simulink model "HW1_MealyV2"  (R2017a)
settings: Solver=VariableStepAuto  StartTime=0.0  StopTime=inf  RelTol=1e-3
settings Model: Creator=avise  LastModifiedBy=nauga

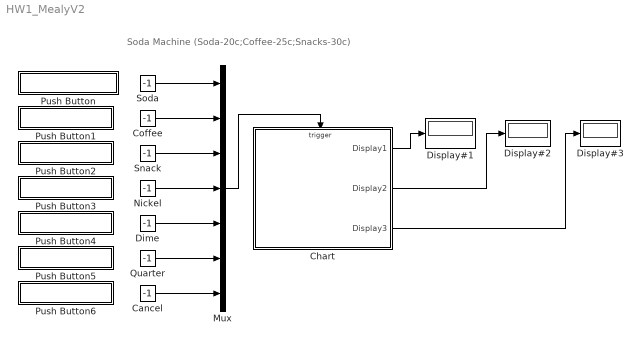
== system HW1_MealyV2 ==
  note: Soda Machine
      | (Soda-20c;Coffee-25c;Snacks-30c)
  Cancel : Constant  Value=-1
  Chart : Stateflow chart  TreatAsAtomicUnit=on
  Coffee : Constant  Value=-1
  Dime : Constant  Value=-1
  Display#1 : Display
  Display#2 : Display
  Display#3 : Display
  Mux : Mux  Inputs=7
  Nickel : Constant  Value=-1
  Push Button : Subsystem  DialogController=hmiCreateDDGDialog  IsWebBlock=on  mask(MWDashboardBlock){webBlockId=664f21db-061d-45c4-a5ed-301e6e3db717, webBlockType=pushbutton, ShowInLibBrwoser=on, ShowInitialText=on, HMISrcModelName=HW1_MealyV2}
      mask prompts: webBlockId "WebBlock Id"; webBlockType "WebBlock Type"; HMISrcModelName "Source Model"
      mask help: SimulinkHMI:dialogs:PushButtonDialogDesc
      mask Help: helpview([docroot '/mapfiles/simulink.map'], 'hmi_push_button')
      mask Display:
      | model = bdroot(gcb);
      | if strcmp(get_param(model,'BlockDiagramType'), 'library')
      |     image([(matlabroot) '/toolbox/simulink/hmi/icons/PushButton.png']);
      | end
  Push Button1 : Subsystem  DialogController=hmiCreateDDGDialog  IsWebBlock=on  mask(MWDashboardBlock){webBlockId=369ec6e0-de46-472e-8dd1-8918505b40b8, webBlockType=pushbutton, ShowInLibBrwoser=on, ShowInitialText=on, HMISrcModelName=HW1_MealyV2}
      mask prompts: webBlockId "WebBlock Id"; webBlockType "WebBlock Type"; HMISrcModelName "Source Model"
      mask help: SimulinkHMI:dialogs:PushButtonDialogDesc
      mask Help: helpview([docroot '/mapfiles/simulink.map'], 'hmi_push_button')
      mask Display:
      | model = bdroot(gcb);
      | if strcmp(get_param(model,'BlockDiagramType'), 'library')
      |     image([(matlabroot) '/toolbox/simulink/hmi/icons/PushButton.png']);
      | end
  Push Button2 : Subsystem  DialogController=hmiCreateDDGDialog  IsWebBlock=on  mask(MWDashboardBlock){webBlockId=437ecff1-f85d-43e6-a183-e5cb8b815949, webBlockType=pushbutton, ShowInLibBrwoser=on, ShowInitialText=on, HMISrcModelName=HW1_MealyV2}
      mask prompts: webBlockId "WebBlock Id"; webBlockType "WebBlock Type"; HMISrcModelName "Source Model"
      mask help: SimulinkHMI:dialogs:PushButtonDialogDesc
      mask Help: helpview([docroot '/mapfiles/simulink.map'], 'hmi_push_button')
      mask Display:
      | model = bdroot(gcb);
      | if strcmp(get_param(model,'BlockDiagramType'), 'library')
      |     image([(matlabroot) '/toolbox/simulink/hmi/icons/PushButton.png']);
      | end
  Push Button3 : Subsystem  DialogController=hmiCreateDDGDialog  IsWebBlock=on  mask(MWDashboardBlock){webBlockId=f2e822cd-a8a7-4ab8-9e8e-7b39c5c413d8, webBlockType=pushbutton, ShowInLibBrwoser=on, ShowInitialText=on, HMISrcModelName=HW1_MealyV2}
      mask prompts: webBlockId "WebBlock Id"; webBlockType "WebBlock Type"; HMISrcModelName "Source Model"
      mask help: SimulinkHMI:dialogs:PushButtonDialogDesc
      mask Help: helpview([docroot '/mapfiles/simulink.map'], 'hmi_push_button')
      mask Display:
      | model = bdroot(gcb);
      | if strcmp(get_param(model,'BlockDiagramType'), 'library')
      |     image([(matlabroot) '/toolbox/simulink/hmi/icons/PushButton.png']);
      | end
  Push Button4 : Subsystem  DialogController=hmiCreateDDGDialog  IsWebBlock=on  mask(MWDashboardBlock){webBlockId=f0c8a644-454f-4bf4-a778-a88d9125c533, webBlockType=pushbutton, ShowInLibBrwoser=on, ShowInitialText=on, HMISrcModelName=HW1_MealyV2}
      mask prompts: webBlockId "WebBlock Id"; webBlockType "WebBlock Type"; HMISrcModelName "Source Model"
      mask help: SimulinkHMI:dialogs:PushButtonDialogDesc
      mask Help: helpview([docroot '/mapfiles/simulink.map'], 'hmi_push_button')
      mask Display:
      | model = bdroot(gcb);
      | if strcmp(get_param(model,'BlockDiagramType'), 'library')
      |     image([(matlabroot) '/toolbox/simulink/hmi/icons/PushButton.png']);
      | end
  Push Button5 : Subsystem  DialogController=hmiCreateDDGDialog  IsWebBlock=on  mask(MWDashboardBlock){webBlockId=21d649ba-39b7-4048-9903-c8ade3fb44d4, webBlockType=pushbutton, ShowInLibBrwoser=on, ShowInitialText=on, HMISrcModelName=HW1_MealyV2}
      mask prompts: webBlockId "WebBlock Id"; webBlockType "WebBlock Type"; HMISrcModelName "Source Model"
      mask help: SimulinkHMI:dialogs:PushButtonDialogDesc
      mask Help: helpview([docroot '/mapfiles/simulink.map'], 'hmi_push_button')
      mask Display:
      | model = bdroot(gcb);
      | if strcmp(get_param(model,'BlockDiagramType'), 'library')
      |     image([(matlabroot) '/toolbox/simulink/hmi/icons/PushButton.png']);
      | end
  Push Button6 : Subsystem  DialogController=hmiCreateDDGDialog  IsWebBlock=on  mask(MWDashboardBlock){webBlockId=33373d40-ddda-4141-b1fc-f71dcaba8225, webBlockType=pushbutton, ShowInLibBrwoser=on, ShowInitialText=on, HMISrcModelName=HW1_MealyV2}
      mask prompts: webBlockId "WebBlock Id"; webBlockType "WebBlock Type"; HMISrcModelName "Source Model"
      mask help: SimulinkHMI:dialogs:PushButtonDialogDesc
      mask Help: helpview([docroot '/mapfiles/simulink.map'], 'hmi_push_button')
      mask Display:
      | model = bdroot(gcb);
      | if strcmp(get_param(model,'BlockDiagramType'), 'library')
      |     image([(matlabroot) '/toolbox/simulink/hmi/icons/PushButton.png']);
      | end
  Quarter : Constant  Value=-1
  Snack : Constant  Value=-1
  Soda : Constant  Value=-1
  wires:
  Cancel/1 -> Mux/7
  Snack/1 -> Mux/3
  Soda/1 -> Mux/1
  Coffee/1 -> Mux/2
  Chart/1(Display1) -> Display#1/1
  Mux/1 -> Chart/Trigger
  Quarter/1 -> Mux/6
  Dime/1 -> Mux/5
  Nickel/1 -> Mux/4
  Chart/2(Display2) -> Display#2/1
  Chart/3(Display3) -> Display#3/1

== system HW1_MealyV2/Push Button ==

== system HW1_MealyV2/Push Button1 ==

== system HW1_MealyV2/Push Button2 ==

== system HW1_MealyV2/Push Button3 ==

== system HW1_MealyV2/Push Button4 ==

== system HW1_MealyV2/Push Button5 ==

== system HW1_MealyV2/Push Button6 ==

== stateflow chart HW1_MealyV2/Chart ==
  state SodaCycle
    state FiveCents
    state TenCents
    state FifteenCents
    state TwentyCents
      en:Reset
    FiveCents -> TwentyCents [order 3] : Quarter{Display1=0;Display2=0;Display3=10;}
    TenCents -> TwentyCents [order 3] : Quarter{Display1=0;Display2=0;Display3=15}
    FiveCents -> FifteenCents [order 2] : Dime{Display1=1;Display2=15}
    TenCents -> FifteenCents [order 1] : Nickel{Display1=1;Display2=15}
    FifteenCents -> TwentyCents [order 1] : Nickel{Display1=0;Display2=0;Display3=0}
    FiveCents -> TenCents [order 1] : Nickel{Display1=1;Display2=10}
    FifteenCents -> TwentyCents [order 3] : Quarter{Display1=0;Display2=0;Display3=20;}
    FiveCents -> FiveCents [order 4] : Coffee|Snack{Display1=9;}
    FiveCents -> (junction 155) [order 5] : Cancel{Display1=0;Display2=0;Display3=5}
    TenCents -> TenCents [order 4] : Coffee|Snack{Display1=9}
    TenCents -> (junction 155) [order 5] : Cancel{Display1=0;Display2=0;Display3=10}
    TenCents -> TwentyCents [order 2] : Dime{Display1=0;Display2=0;Display3=0}
    FifteenCents -> TwentyCents [order 2] : Dime{Display1=0;Display2=0;Display3=5}
    FifteenCents -> (junction 155) [order 5] : Cancel{Display1=0;Display2=0;Display3=15}
    FifteenCents -> FifteenCents [order 4] : Coffee|Snack{Display1=9}
  state Soda
    %20c
  state Wait
  state CoffeeCycle
    state Five
    state Fifteen
    state Twenty
    state TwentyFive
      en:Reset
    state Ten
    CoffeeCycle.Five -> CoffeeCycle.TwentyFive [order 3] : Quarter{Display1=0;Display2=0;Display3=5}
    CoffeeCycle.Ten -> CoffeeCycle.Twenty [order 2] : Dime{Display1=2;Display2=20}
    CoffeeCycle.Fifteen -> CoffeeCycle.TwentyFive [order 4] : Quarter{Display1=0;Display2=0;Display3=15}
    CoffeeCycle.Fifteen -> CoffeeCycle.TwentyFive [order 3] : Dime{Display1=0;Display2=0;Display3=0}
    CoffeeCycle.Five -> CoffeeCycle.Fifteen [order 2] : Dime{Display1=2;Display2=15}
    CoffeeCycle.Five -> CoffeeCycle.Five [order 4] : Soda|Snack{Display1=9}
    CoffeeCycle.Twenty -> CoffeeCycle.Twenty [order 4] : Soda|Snack{Display1=9}
    CoffeeCycle.Fifteen -> CoffeeCycle.Fifteen [order 2] : Soda|Snack{Display1=9}
    CoffeeCycle.Ten -> CoffeeCycle.Ten [order 4] : Soda|Snack{Display1=9}
    CoffeeCycle.Ten -> CoffeeCycle.TwentyFive [order 3] : Quarter{Display1=0;Display2=0;Display3=10}
    CoffeeCycle.Five -> CoffeeCycle.Ten [order 1] : Nickel{Display1=2;Display2=10}
    CoffeeCycle.Fifteen -> CoffeeCycle.Twenty [order 1] : Nickel{Display1=2;Display2=20}
    CoffeeCycle.Ten -> CoffeeCycle.Fifteen [order 1] : Nickel{Display1=2;Display2=15}
    CoffeeCycle.Twenty -> CoffeeCycle.TwentyFive [order 1] : Nickel{Display1=0;Display2=0;Display3=0}
    CoffeeCycle.Five -> (junction 195) [order 5] : Cancel{Display1=0;Display2=0;Display3=5}
    CoffeeCycle.Ten -> (junction 195) [order 5] : Cancel{Display1=0;Display2=0;Display3=10}
    CoffeeCycle.Fifteen -> (junction 195) [order 5] : Cancel{Display1=0;Display2=0;Display3=15}
    CoffeeCycle.Twenty -> (junction 195) [order 5] : Cancel{Display1=0;Display2=0;Display3=20}
    CoffeeCycle.Twenty -> CoffeeCycle.TwentyFive [order 3] : Quarter{Display1=0;Display2=0;Display3=20}
    CoffeeCycle.Twenty -> CoffeeCycle.TwentyFive [order 2] : Dime{Display1=0;Display2=0;Display3=5}
  state Coffee
    %25c
  state SnackCycle
    state Twenty
    state TwentyFive
    state Five
    state Ten
    state Fifteen
    state Thirty
      en:Reset
    SnackCycle.Five -> Thirty [order 3] : Quarter{Display1=0;Display2=0;Display3=0}
    SnackCycle.TwentyFive -> Thirty [order 4] : Quarter{Display1=0;Display2=0;Display3=20}
    SnackCycle.Ten -> Thirty [order 4] : Quarter{Display1=0;Display2=0;Display3=5}
    SnackCycle.Fifteen -> Thirty [order 4] : Quarter{Display1=0;Display2=0;Display3=10}
    SnackCycle.Fifteen -> SnackCycle.TwentyFive [order 3] : Dime{Display1=3;Display2=25}
    SnackCycle.Ten -> SnackCycle.Twenty [order 3] : Dime{Display1=3;Display2=20}
    SnackCycle.Twenty -> Thirty [order 4] : Quarter{Display1=0;Display2=0;Display3=15}
    SnackCycle.Five -> SnackCycle.Fifteen [order 2] : Dime{Display1=3;Display2=15}
    SnackCycle.Twenty -> Thirty [order 3] : Dime{Display1=0;Display2=0;Display3=0}
    SnackCycle.Five -> SnackCycle.Ten [order 1] : Nickel{Display1=3;Display2=10}
    SnackCycle.Ten -> SnackCycle.Fifteen [order 2] : Nickel{Display1=3;Display2=15}
    SnackCycle.Twenty -> SnackCycle.TwentyFive [order 2] : Nickel{Display1=3;Display2=25}
    SnackCycle.Fifteen -> SnackCycle.Twenty [order 2] : Nickel{Display1=3;Display2=20}
    SnackCycle.TwentyFive -> Thirty [order 2] : Nickel{Display1=0;Display2=0;Display3=0}
    SnackCycle.TwentyFive -> Thirty [order 3] : Dime{Display1=0;Display2=0;Display3=5}
    SnackCycle.Five -> SnackCycle.Five [order 4] : Soda|Coffee{Display1=9}
    SnackCycle.Five -> (junction 243) [order 5] : Cancel{Display1=0;Display2=0;Display3=5}
    SnackCycle.Ten -> SnackCycle.Ten [order 1] : Soda|Coffee{Display1=9}
    SnackCycle.Ten -> (junction 243) [order 5] : Cancel{Display1=0;Display2=0;Display3=10}
    SnackCycle.Fifteen -> SnackCycle.Fifteen [order 1] : Soda|Coffee{Display1=9}
    SnackCycle.Fifteen -> (junction 243) [order 5] : Cancel{Display1=0;Display2=0;Display3=15}
    SnackCycle.TwentyFive -> (junction 243) [order 5] : Cancel{Display1=0;Display2=0;Display3=25}
    SnackCycle.TwentyFive -> SnackCycle.TwentyFive [order 1] : Soda|Coffee{Display1=9}
    SnackCycle.Twenty -> (junction 243) [order 5] : Cancel{Display1=0;Display2=0;Display3=20}
    SnackCycle.Twenty -> SnackCycle.Twenty [order 1] : Soda|Coffee{Display1=9}
  state Snack
    %30c
  (default) -> Wait
  TwentyCents -> Wait : Reset
  Wait -> Wait [order 4] : Quarter{Display3=25;}
  Soda -> FiveCents [order 1] : Nickel{Display2=5}
  Wait -> Soda [order 6] : Soda{Display1=1;
      | Display3=-1;}
  Thirty -> Wait : Reset
  Soda -> TwentyCents [order 3] : Quarter{Display1=0;Display2=0;Display3=5}
  Soda -> TenCents [order 2] : Dime{Display2=10}
  (junction 243) -> Wait
  (junction 195) -> Wait
  Wait -> Snack [order 7] : Snack{Display1=3;
      | Display3=-1;}
  CoffeeCycle.TwentyFive -> Wait : Reset
  Wait -> Wait [order 3] : Nickel{Display3=5;}
  Wait -> Coffee [order 2] : Coffee{Display1=2;
      | Display3=-1;}
  Wait -> Wait [order 1] : Dime{Display3=10;}
  Wait -> Wait [order 5] : Cancel
  (junction 155) -> Wait
  Coffee -> CoffeeCycle.Five [order 1] : Nickel{Display2=5}
  Coffee -> CoffeeCycle.Ten [order 2] : Dime{Display2=10}
  Coffee -> CoffeeCycle.TwentyFive [order 3] : Quarter{Display1=0;Display2=0;Display3=0}
  Snack -> SnackCycle.Five [order 1] : Nickel{Display2=5}
  Snack -> SnackCycle.TwentyFive [order 3] : Quarter{Display2=25}
  Snack -> SnackCycle.Ten [order 2] : Dime{Display2=10}
  data: Display1 output =0; Display2 output =0; Display3 output =-1
  events: Soda input EITHER_EDGE_EVENT; Coffee input EITHER_EDGE_EVENT; Snack input EITHER_EDGE_EVENT; Nickel input RISING_EDGE_EVENT; Dime input RISING_EDGE_EVENT; Quarter input RISING_EDGE_EVENT; Cancel input EITHER_EDGE_EVENT; Reset local FUNCTION_CALL_EVENT
